simulink model "Ex_03_I_Control_Plus_Feedforward"  (Simulink 8.9)
settings: Solver=ode3  StartTime=0.0  StopTime=t_max  FixedStep=jointObj.Ts  RelTol=1e-3
values from neighbouring files (symbols this model uses):
  t_max = f_max    (= 100)    [Ex_00_example_config.m]
libraries: simulink x1, cjt_library_controllers x1, cjt_library_models x1
settings Model: SuppressorTable=22 serialization::archive 11 0 6 0 0 0 11 0  Creator=joern  LastModifiedBy=wesley
settings DataIOCC: LimitDataPoints=off  SignalLoggingSaveFormat=Dataset
settings DebuggingCC: UnderspecifiedInitializationDetection=Simplified  MergeDetectMultiDrivingBlocksExec=error  SolverPrmCheckMsg=warning  FcnCallInpInsideContextMsg=error  StateNameClashWarn=none
settings GRTTargetCC: CombineOutputUpdateFcns=on  GRTInterface=off
settings ConfigComp: CovSFcnEnable=off

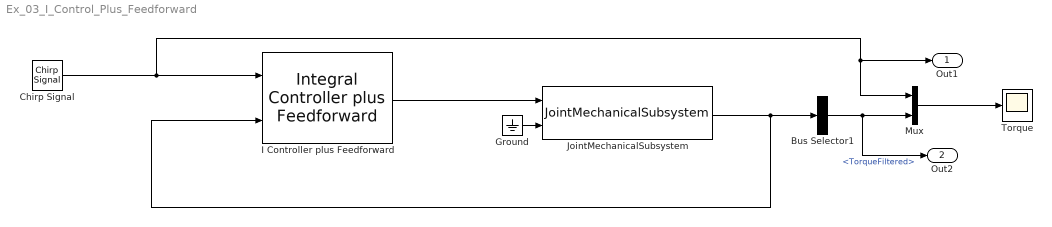
== system Ex_03_I_Control_Plus_Feedforward ==
  Bus Selector1 : BusSelector  OutputSignals=TorqueFiltered
  Chirp Signal : simulink/Sources/Chirp Signal  f1=f_min  T=t_max  f2=f_max
  Ground : Ground
  I Controller plus Feedforward : cjt_library_controllers/Controllers/Integral Controller plus Feedforward  jointObj=jointObj  I_Gain=10
  JointMechanicalSubsystem : cjt_library_models/Joint models/JointMechanicalSubsystem  jointObj=jointObj  fc_vel=499  fc_torque=499  input_delay=1  output_delay=1  quantize=on  quantize_bits=19  input_noise_enabled=off  output_noise_enabled=off  var_u=0.12^2  var_y=1.8e-10
  Mux : Mux  Inputs=2
  Torque : Scope
  Out1 : Outport  SignalName=Reference
  Out2 : Outport  Port=2  SignalName=Response
  wires:
  Mux/1 -> Torque/1
  Ground/1 -> JointMechanicalSubsystem/2
  JointMechanicalSubsystem/1 -> I Controller plus Feedforward/2, Bus Selector1/1
  I Controller plus Feedforward/1 -> JointMechanicalSubsystem/1
  Chirp Signal/1 -> I Controller plus Feedforward/1, Out1/1, Mux/1
  Bus Selector1/1 -> Out2/1, Mux/2  "<TorqueFiltered>"
